simulink model "fuzzy_simulator_intellihire"  (R2016a)
settings: Solver=FixedStepAuto  SolverMode=SingleTasking  StartTime=0.0  StopTime=13891  FixedStep=1  RelTol=1e-3
libraries: fuzblock x1
settings Model: Creator=caxenie  LastModifiedBy=caxenie
settings DataIOCC: LimitDataPoints=on  SaveOutput=off  SaveTime=off
settings OptimizationCC: BlockReduction=off  BooleanDataType=off
settings DebuggingCC: SaveWithParameterizedLinksMsg=none  UnderspecifiedInitializationDetection=Classic  MergeDetectMultiDrivingBlocksExec=none  SignalResolutionControl=TryResolveAllWithWarning  AllowSymbolicDim=off
settings HardwareCC: TargetUnknown=on

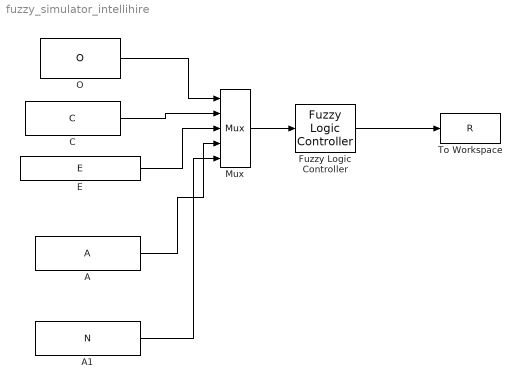
== system fuzzy_simulator_intellihire ==
  A : FromWorkspace  VariableName=A  SampleTime=0
  A1 : FromWorkspace  VariableName=N  SampleTime=0
  C : FromWorkspace  VariableName=C  SampleTime=0
  E : FromWorkspace  VariableName=E  SampleTime=0
  Fuzzy Logic Controller : fuzblock/Fuzzy Logic  Controller  fis=fuzzy_inference_system_mamdani
  Mux : Mux  Inputs=5
  O : FromWorkspace  VariableName=O  SampleTime=0
  To Workspace : ToWorkspace  VariableName=R  SaveFormat=Timeseries  SampleTime=-1
  wires:
  C/1 -> Mux/2
  O/1 -> Mux/1
  E/1 -> Mux/3
  A/1 -> Mux/4
  Mux/1 -> Fuzzy Logic Controller/1
  Fuzzy Logic Controller/1 -> To Workspace/1
  A1/1 -> Mux/5
